simulink model "sampleModel1623"  (R2023a)
settings: Solver=VariableStepAuto  StartTime=0.0  StopTime=10.0  RelTol=1e-3
libraries: simulink x4, hdlsllib x2
settings Model: Creator=user1  LastModifiedBy=user1

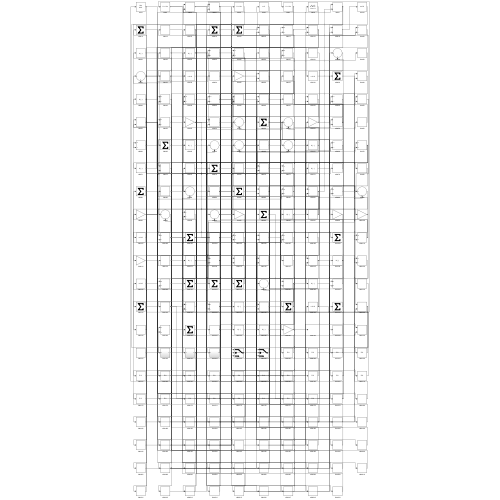
[thumbnail: Simulink's stored preview of the top-level diagram]
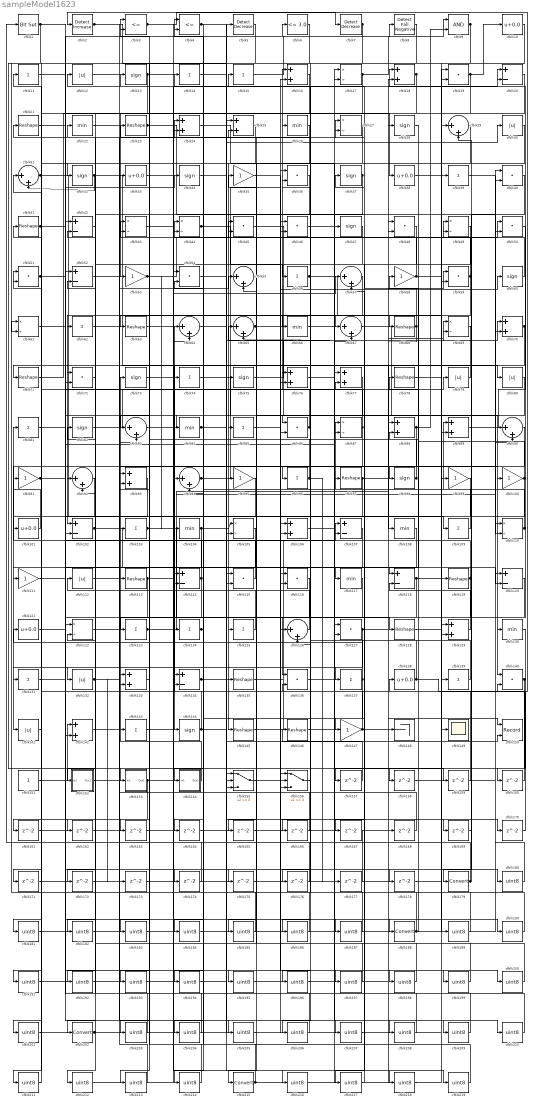
== system sampleModel1623 ==
  cfblk1 : simulink/Logic and Bit Operations/Bit Set  iBit=0
      settings: LibrarySourceBlock=|
      | hdlsllib/Logic and Bit
      | Operations/Bit Set
  cfblk{10,33,38,101,121,138} (6 alike) : Bias  Bias=0.0  SaturateOnIntegerOverflow=off
  cfblk{35,53,58,91,95,99..100,111,147} (9 alike) : Gain
  cfblk{20,42,52,102,107,114,118,120,134} (9 alike) : Sum  Inputs=+-
  cfblk{11,14..15,39,56,62,74,81,85,96,103,109,123..125,131,137,139,143} (19 alike) : Sum  Inputs=+
  cfblk{22,26,66,84,104,108,117,130} (8 alike) : MinMax
  cfblk{17,27,43..44,49,61,69,87,105,110,122} (11 alike) : Product  Inputs=*/  RndMeth=Zero  SaturateOnIntegerOverflow=on
  cfblk{16,18,24..25,70,76..77,88..89,93,106,129,133,142} (14 alike) : Sum
  cfblk{12,30,79..80,112,132,141} (7 alike) : Abs  SaturateOnIntegerOverflow=off
  cfblk{21,23,41,63,68,71,78,97,113,119,128,135,145..146} (14 alike) : Reshape
  cfblk{19,36,40,45..46,48,50..51,54,59,72,86,115..116,127,136,140} (17 alike) : DotProduct  OutDataTypeStr=Inherit: Inherit via internal rule
  cfblk{29,31,55,57,64..65,67,83,90,92,94,126} (12 alike) : Sum  Inputs=|++
  cfblk{13,28,32,34,37,47,60,73,75,82,98,144} (12 alike) : Signum
  cfblk148 : Terminator
  cfblk149 : Scope
  cfblk150 : Record  FileSettingsInternal="{\"entries\":[{\"content\":{\"excelSettings\":{\"content\":{},\"type\":\"Streamout.ExcelSettings\"}},\"type\":\"Streamout.FileSettingStorage\",\"uuid\":\"\"}],\"packageUris\":[\"http:\\/\\/schema.mathworks.com\\/mf0\\/streamout_blocks\\/R2020a\"],\"version\":\"1.0\"}"  Layout=[1 1]  SignalsInternal="{\"entries\":[{\"content\":{\"signals\":[{\"content\":{\"blockPath\":[],\"dimensions\":[1],\"domain\":\"\",\"lineColor\":\"#a2142f\",\"plots\":[1],\"port\":1,\"signalID\":2350,\"signalName\":\"XY Graph:1\"},\"type\":\"RecordBlkView.Signal\",\"uuid\":\"\"},{\"content\":{\"blockPath\":[],\"dimensions\":[1],\"domain\":\"\",\"lineColor\":\"#139fff\",\"plots\":[1],\"port\":2,\"signalID\":2353,\"signalName\":\"XY Graph:2\"},\"type\":\"RecordBlkView.Signal\",\"uuid\":\"\"}]},\"type\":\"RecordBlkView.InputSignals\",\"uuid\":\"\"}],\"packageUris\":[\"http:\\/\\/schema.mathworks.com\\/mf0\\/streamout_blocks\\/R2020a\"],\"version\":\"1.0\"}"  VisualizationBindings="{\"xyplotplugin\":{\"info\":[{\"series\":[{\"bindingParametersList\":[{\"parameter\":\"X-Axis\",\"signalID\":2350,\"signalName\":\"XY Graph:1\"},{\"parameter\":\"Y-Axis\",\"signalID\":2353,\"signalName\":\"XY Graph:2\"}],\"seriesID\":37193}],\"subplotID\":1}]}}"  CompatibilityTag=XY  st=-1
  cfblk151 : Constant  SampleTime=-1
  cfblk152 : Subsystem
      settings: LibrarySourceBlock=|
      | hdlsllib/Ports &
      | Subsystems/Subsystem
  cfblk153 : Subsystem
      settings: LibrarySourceBlock=|
      | hdlsllib/Ports &
      | Subsystems/Subsystem
  cfblk154 : Subsystem
      settings: LibrarySourceBlock=|
      | hdlsllib/Ports &
      | Subsystems/Subsystem
  cfblk155 : Switch  SaturateOnIntegerOverflow=off  InputSameDT=off
  cfblk156 : Switch  SaturateOnIntegerOverflow=off  InputSameDT=off
  cfblk{157..178} (22 alike) : Delay  SampleTime=1
  cfblk{179,188,202,215} (4 alike) : DataTypeConversion  SaturateOnIntegerOverflow=off  RndMeth=Floor
  cfblk{180..187,189..201,203..214,216..219} (37 alike) : DataTypeConversion  OutDataTypeStr=uint8  SaturateOnIntegerOverflow=off  RndMeth=Floor
  cfblk2 : simulink/Logic and Bit Operations/Detect Increase  vinit=0.0  OutDataTypeStr=boolean
      settings: LibrarySourceBlock=|
      | hdlsllib/Logic and Bit
      | Operations/Detect
      | Increase
  cfblk3 : RelationalOperator  Operator=<=  OutDataTypeStr=boolean  InputSameDT=off
  cfblk4 : RelationalOperator  Operator=<=  OutDataTypeStr=boolean  InputSameDT=off
  cfblk5 : simulink/Logic and Bit Operations/Detect Decrease  vinit=0.0  OutDataTypeStr=boolean
      settings: LibrarySourceBlock=|
      | hdlsllib/Logic and Bit
      | Operations/Detect
      | Decrease
  cfblk6 : hdlsllib/Logic and Bit Operations/Compare To Constant  relop=<=  const=3.0  OutDataTypeStr=boolean
  cfblk7 : simulink/Logic and Bit Operations/Detect Decrease  vinit=0.0  OutDataTypeStr=boolean
      settings: LibrarySourceBlock=|
      | hdlsllib/Logic and Bit
      | Operations/Detect
      | Decrease
  cfblk8 : hdlsllib/Logic and Bit Operations/Detect Fall Negative  vinit=0  OutDataTypeStr=boolean
  cfblk9 : Logic  AllPortsSameDT=off  OutDataTypeStr=boolean
  wires:
  cfblk119/1 -> cfblk92/2, cfblk206/1
  cfblk71/1 -> cfblk38/1
  cfblk144/1 -> cfblk64/1, cfblk150/2
  cfblk83/1 -> cfblk86/1
  cfblk154/1(Out1) -> cfblk73/1
  cfblk65/1 -> cfblk80/1, cfblk200/1
  cfblk25/1 -> cfblk145/1
  cfblk98/1 -> cfblk21/1, cfblk24/1
  cfblk32/1 -> cfblk144/1, cfblk31/2
  cfblk89/1 -> cfblk18/1
  cfblk60/1 -> cfblk49/1
  cfblk1/1 -> cfblk153/1(In1), cfblk90/2
  cfblk57/1 -> cfblk102/1
  cfblk30/1 -> cfblk98/1
  cfblk92/1 -> cfblk141/1
  cfblk114/1 -> cfblk81/1, cfblk192/1
  cfblk15/1 -> cfblk8/1
  cfblk28/1 -> cfblk118/1
  cfblk61/1 -> cfblk102/2
  cfblk146/1 -> cfblk188/1
  cfblk31/1 -> cfblk109/1, cfblk105/2
  cfblk109/1 -> cfblk89/1
  cfblk53/1 -> cfblk50/1, cfblk104/1, cfblk106/2
  cfblk19/1 -> cfblk53/1, cfblk10/1
  cfblk67/1 -> cfblk140/1
  cfblk151/1 -> cfblk142/1
  cfblk51/1 -> cfblk120/2, cfblk174/1, cfblk175/1
  cfblk40/1 -> cfblk179/1
  cfblk52/1 -> cfblk67/1
  cfblk66/1 -> cfblk128/1
  cfblk127/1 -> cfblk137/1, cfblk69/2, cfblk181/1
  cfblk10/1 -> cfblk33/1
  cfblk68/1 -> cfblk15/1, cfblk65/2
  cfblk108/1 -> cfblk154/1(In1)
  cfblk82/1 -> cfblk16/1
  cfblk62/1 -> cfblk108/1
  cfblk107/1 -> cfblk117/1
  cfblk97/1 -> cfblk59/1, cfblk183/1
  cfblk59/1 -> cfblk43/1, cfblk27/2, cfblk166/1
  cfblk26/1 -> cfblk71/1
  cfblk75/1 -> cfblk69/1
  cfblk104/1 -> cfblk105/1, cfblk191/1
  cfblk79/1 -> cfblk72/1
  cfblk54/1 -> cfblk135/1
  cfblk139/1 -> cfblk23/1
  cfblk125/1 -> cfblk82/1
  cfblk145/1 -> cfblk17/1
  cfblk106/1 -> cfblk47/1
  cfblk24/1 -> cfblk127/1
  cfblk118/1 -> cfblk129/1, cfblk142/2, cfblk58/1
  cfblk37/1 -> cfblk62/1, cfblk114/1, cfblk193/1
  cfblk135/1 -> cfblk107/1
  cfblk39/1 -> cfblk50/2
  cfblk147/1 -> cfblk113/1, cfblk150/1
  cfblk137/1 -> cfblk121/1, cfblk12/1, cfblk184/1
  cfblk90/1 -> cfblk101/1
  cfblk47/1 -> cfblk92/1
  cfblk117/1 -> cfblk136/1
  cfblk112/1 -> cfblk79/1
  cfblk94/1 -> cfblk16/2, cfblk100/1
  cfblk113/1 -> cfblk123/1, cfblk20/2
  cfblk95/1 -> cfblk134/1
  cfblk133/1 -> cfblk3/1
  cfblk56/1 -> cfblk139/1, cfblk99/1
  cfblk12/1 -> cfblk96/1
  cfblk34/1 -> cfblk26/1
  cfblk49/1 -> cfblk147/1
  cfblk110/1 -> cfblk44/1, cfblk87/1
  cfblk84/1 -> cfblk30/1, cfblk169/1
  cfblk45/1 -> cfblk110/2
  cfblk23/1 -> cfblk90/1, cfblk64/2
  cfblk78/1 -> cfblk39/1
  cfblk63/1 -> cfblk85/1
  cfblk77/1 -> cfblk215/1
  cfblk2/1 -> cfblk95/1, cfblk127/2
  cfblk87/1 -> cfblk152/1(In1), cfblk4/2
  cfblk126/1 -> cfblk52/2
  cfblk91/1 -> cfblk34/1, cfblk74/1, cfblk87/2
  cfblk42/1 -> cfblk202/1
  cfblk18/1 -> cfblk63/1, cfblk114/2
  cfblk105/1 -> cfblk111/1
  cfblk85/1 -> cfblk60/1
  cfblk55/1 -> cfblk25/2
  cfblk70/1 -> cfblk76/2, cfblk171/1, cfblk172/1
  cfblk152/1(Out1) -> cfblk55/1
  cfblk8/1 -> cfblk131/1
  cfblk141/1 -> cfblk41/1
  cfblk123/1 -> cfblk28/1, cfblk103/1
  cfblk13/1 -> cfblk134/2, cfblk132/1, cfblk72/2
  cfblk101/1 -> cfblk91/1
  cfblk50/1 -> cfblk130/1
  cfblk41/1 -> cfblk6/1, cfblk211/1
  cfblk132/1 -> cfblk83/2, cfblk173/1
  cfblk9/1 -> cfblk59/2, cfblk66/1
  cfblk138/1 -> cfblk2/1, cfblk65/1, cfblk57/2
  cfblk115/1 -> cfblk94/2
  cfblk4/1 -> cfblk68/1, cfblk204/1
  cfblk3/1 -> cfblk7/1, cfblk75/1
  cfblk121/1 -> cfblk76/1
  cfblk88/1 -> cfblk9/2, cfblk196/1
  cfblk129/1 -> cfblk88/2
  cfblk142/1 -> cfblk27/1
  cfblk102/1 -> cfblk124/1, cfblk156/3
  cfblk7/1 -> cfblk56/1, cfblk61/2
  cfblk96/1 -> cfblk4/1, cfblk177/1
  cfblk74/1 -> cfblk156/1
  cfblk100/1 -> cfblk125/1, cfblk78/1
  cfblk103/1 -> cfblk156/2, cfblk70/2
  cfblk153/1(Out1) -> cfblk45/1, cfblk57/1, cfblk201/1
  cfblk44/1 -> cfblk126/1, cfblk86/2
  cfblk58/1 -> cfblk37/1, cfblk20/1
  cfblk38/1 -> cfblk149/1
  cfblk17/1 -> cfblk32/1, cfblk9/1, cfblk83/1
  cfblk20/1 -> cfblk115/2
  cfblk156/1 -> cfblk136/2
  cfblk140/1 -> cfblk133/2, cfblk157/1
  cfblk124/1 -> cfblk14/1, cfblk214/1
  cfblk86/1 -> cfblk51/1, cfblk51/2, cfblk176/1
  cfblk134/1 -> cfblk70/1, cfblk170/1
  cfblk111/1 -> cfblk107/2
  cfblk157/1 -> cfblk126/2
  cfblk136/1 -> cfblk158/1
  cfblk158/1 -> cfblk110/1
  cfblk64/1 -> cfblk159/1
  cfblk159/1 -> cfblk25/1
  cfblk130/1 -> cfblk160/1
  cfblk160/1 -> cfblk31/1
  cfblk16/1 -> cfblk161/1
  cfblk161/1 -> cfblk94/1
  cfblk72/1 -> cfblk162/1
  cfblk162/1 -> cfblk88/1
  cfblk6/1 -> cfblk163/1
  cfblk163/1 -> cfblk3/2
  cfblk5/1 -> cfblk164/1
  cfblk164/1 -> cfblk17/2
  cfblk27/1 -> cfblk165/1
  cfblk165/1 -> cfblk18/2
  cfblk166/1 -> cfblk45/2
  cfblk120/1 -> cfblk167/1
  cfblk167/1 -> cfblk1/1
  cfblk168/1 -> cfblk133/1
  cfblk169/1 -> cfblk49/2
  cfblk170/1 -> cfblk140/2
  cfblk171/1 -> cfblk129/2
  cfblk172/1 -> cfblk67/2
  cfblk173/1 -> cfblk89/2
  cfblk174/1 -> cfblk52/1
  cfblk175/1 -> cfblk55/2
  cfblk176/1 -> cfblk24/2
  cfblk177/1 -> cfblk44/2
  cfblk73/1 -> cfblk178/1
  cfblk178/1 -> cfblk118/2
  cfblk179/1 -> cfblk29/2, cfblk106/1
  cfblk131/1 -> cfblk180/1
  cfblk180/1 -> cfblk40/1
  cfblk181/1 -> cfblk40/2
  cfblk116/1 -> cfblk182/1
  cfblk182/1 -> cfblk120/1
  cfblk183/1 -> cfblk116/1
  cfblk184/1 -> cfblk116/2
  cfblk36/1 -> cfblk185/1
  cfblk185/1 -> cfblk61/1
  cfblk80/1 -> cfblk186/1
  cfblk186/1 -> cfblk36/1
  cfblk81/1 -> cfblk187/1
  cfblk187/1 -> cfblk36/2
  cfblk188/1 -> cfblk138/1, cfblk84/1
  cfblk128/1 -> cfblk189/1
  cfblk189/1 -> cfblk146/1
  cfblk155/1 -> cfblk190/1
  cfblk190/1 -> cfblk115/1
  cfblk191/1 -> cfblk155/1
  cfblk192/1 -> cfblk155/2
  cfblk193/1 -> cfblk155/3
  cfblk48/1 -> cfblk194/1
  cfblk21/1 -> cfblk195/1
  cfblk195/1 -> cfblk48/1
  cfblk196/1 -> cfblk48/2
  cfblk35/1 -> cfblk197/1
  cfblk197/1 -> cfblk112/1
  cfblk43/1 -> cfblk198/1
  cfblk198/1 -> cfblk35/1
  cfblk46/1 -> cfblk199/1
  cfblk199/1 -> cfblk13/1
  cfblk200/1 -> cfblk46/1
  cfblk201/1 -> cfblk46/2
  cfblk202/1 -> cfblk97/1, cfblk5/1, cfblk148/1
  cfblk29/1 -> cfblk203/1
  cfblk203/1 -> cfblk42/1
  cfblk204/1 -> cfblk42/2
  cfblk22/1 -> cfblk205/1
  cfblk205/1 -> cfblk19/1
  cfblk206/1 -> cfblk22/1
  cfblk122/1 -> cfblk207/1
  cfblk207/1 -> cfblk19/2
  cfblk76/1 -> cfblk208/1
  cfblk208/1 -> cfblk122/1
  cfblk194/1 -> cfblk209/1
  cfblk209/1 -> cfblk122/2
  cfblk11/1 -> cfblk210/1
  cfblk210/1 -> cfblk43/2
  cfblk211/1 -> cfblk11/1
  cfblk93/1 -> cfblk212/1
  cfblk212/1 -> cfblk54/1
  cfblk69/1 -> cfblk213/1
  cfblk213/1 -> cfblk93/1
  cfblk214/1 -> cfblk93/2
  cfblk215/1 -> cfblk168/1, cfblk54/2, cfblk29/1
  cfblk33/1 -> cfblk216/1
  cfblk216/1 -> cfblk77/1
  cfblk99/1 -> cfblk217/1
  cfblk217/1 -> cfblk77/2
  cfblk143/1 -> cfblk218/1
  cfblk218/1 -> cfblk119/1
  cfblk14/1 -> cfblk219/1
  cfblk219/1 -> cfblk143/1

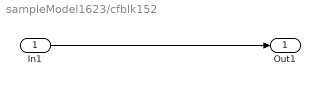
== system sampleModel1623/cfblk152 ==
  In1 : Inport
  Out1 : Outport
  wires:
  In1/1 -> Out1/1

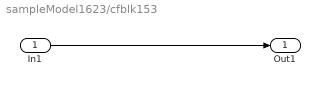
== system sampleModel1623/cfblk153 ==
  In1 : Inport
  Out1 : Outport
  wires:
  In1/1 -> Out1/1

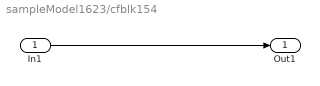
== system sampleModel1623/cfblk154 ==
  In1 : Inport
  Out1 : Outport
  wires:
  In1/1 -> Out1/1
